simulink model "Charge_complete_V2"  (R2020a)
settings: Solver=VariableStepAuto  StartTime=0.0  StopTime=5500  RelTol=1e-3
undefined symbols (not defined in the file): Ion, Lithium
libraries: powerlib x7, electricdrivelib x1
settings Model: Creator=guill  LastModifiedBy=guill

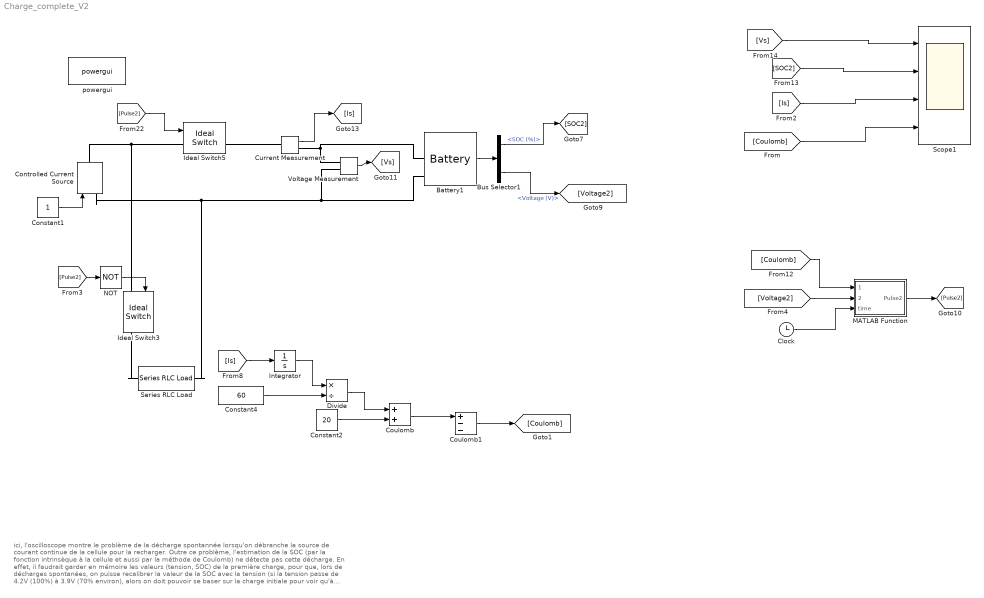
== system Charge_complete_V2 ==
  note: ici, l'oscilloscope montre le problème de la décharge spontannée lorsqu'on débranche la source de courant continue de la cellule pour la recharger. Outre ce problème, l'estimation de la SOC (par la fonction intrinsèque à la cellule et aussi par la méthode de Coulomb) ne détecte pas cette décharge.
      | En effet, il faudrait garder en mémoire les valeurs (tension, SOC) de la première charge, pour que, lors de décharges spontanées, on puisse recalibrer la valeur de la SOC avec la tension (si la tension passe de 4.2V (100%) à 3.9V (70% environ), alors on doit pouvoir se baser sur la charge initiale pour voir qu'à 3.9V, SOC=70%)
  Battery1 : electricdrivelib/Extra Sources/Battery  BatType=Lithium-Ion  ShowTempParam=on  ThermalPreset="3.6V  2.0Ah"  ShowAgeParam=off  NomV=3.5  NomQ=2  SOC=35  Batt_Tr=30  PresetModel=off  MaxQ=2.05  MinV=2.625  FullV=4.1  Dis_rate=0.4  R=0.017  Normal_OP=1.8087  expZone="[3.88         0.2]"  current=[6.5 13 32.5]  Units=Time  Tci=20  NomT=115  T2=0  MaxQ2=1.65  FullV2=4  Normal_OP2=3.25  expZone2="[3.8         0.2]"  Rca=0.06  ti=1000  Dp=0  Neq0=0  Tsim=1e6  Ta1=25  Qeol=5.4*0.9  Reol=0.013333*1.2  Char_age=[2.3478, 3]  Dis_age=[2.3478, 10]  N1=1500  N2=10500  N3=1000  N4=1400  Ta2=45  N5=950
  Bus Selector1 : BusSelector  OutputSignals=SOC (%),Current (A),Voltage (V)
  Clock : Clock
  Constant1 : Constant
  Constant2 : Constant  Value=20
  Constant4 : Constant  Value=60
  Controlled Current Source : powerlib/Electrical Sources/Controlled Current Source  Initialize=on  Source_Type=AC  Amplitude=0  Phase=0  Frequency=0  Measurements=None
  Coulomb : Sum
  Coulomb1 : Sum  Inputs=+--
  Current Measurement : powerlib/Measurements/Current Measurement  PhasorSimulation=off  OutputType=Complex  PSBequivalent=0
  Divide : Product  Inputs=*/
  Ideal Switch3 : powerlib/Power Electronics/Ideal Switch  Ron=0.001  Lon=0  IC=0  Rs=1e5  Cs=inf  Measurements=on
  Ideal Switch5 : powerlib/Power Electronics/Ideal Switch  Ron=0.001  Lon=0  IC=0  Rs=1e5  Cs=inf  Measurements=on
  Integrator : Integrator
  MATLAB Function : MATLAB Function  TreatAsAtomicUnit=on
  NOT : Logic  Operator=NOT  IconShape=distinctive  AllPortsSameDT=off  OutDataTypeStr=boolean
  Scope1 : Scope  NumInputPorts=4
  Series RLC Load : powerlib/Elements/Series RLC Load  LConnTagsString=a  RConnTagsString=__new0  NominalVoltage=10  NominalFrequency=60  ActivePower=1000  InductivePower=0  CapacitivePower=0  Setx0=off  InitialVoltage=0  SetiL0=off  InitialCurrent=0  Measurements=None  LoadType=constant Z
  Voltage Measurement : powerlib/Measurements/Voltage Measurement  PhasorSimulation=off  OutputType=Complex  PSBequivalent=0
  powergui : powerlib/powergui  Priority=1  SimulationMode=Continuous  SampleTime=50e-2  frequency=60  Iterations=50  frequencyindice=0  Pbase=100e6  ErrMax=1e-4  UnitsV=kV  UnitsW=MW  buscounter=0  FunctionMessages=off  echomessages=off  EnableUseOfTLC=off  CurrentSourceSwitches=off  DisableSnubberDevices=off  DisableRonSwitches=off  DisableVfSwitches=off  DisplayEquations=off  AutomaticDiscreteSolvers=off  SolverType=Tustin/Backward Euler (TBE)  Interpol=off  ExternalGateDelay=off  methode=off  Ts=100  x0status=blocks  SPID=on  SwTol=0  HookPort=off  NonlinearTolerance=1e-4  nMaxIteration=100  ContinueOnMaxIteration=off  RestoreLinks=warning  ResistiveCurrentMeasurement=off  Frange=[0:2:500]  Ylog=off  Xlog=on  ShowGrid=off  save=off  variable=ZData  structure=0  ZoomFFT=off  StartTime=0.0  cycles=1  DisplayStyle=1  fundamental=60  FreqAxis=off  MaxFrequency=1000  frequencyindicesteady=1  RmsSteady=1  display=off
  wires:
  [Is] -> Scope1/3
  Coulomb/1 -> Coulomb1/1
  Constant2/1 -> Coulomb/2
  [Pulse2] -> Ideal Switch5/1
  Bus Selector1/1 -> [SOC2]  "<SOC (%)>"
  Integrator/1 -> Divide/1
  Divide/1 -> Coulomb/1
  [SOC2] -> Scope1/2
  Constant1/1 -> Controlled Current Source/1
  NOT/1 -> Ideal Switch3/1
  Battery1/1 -> Bus Selector1/1
  Current Measurement/1 -> [Is]
  Bus Selector1/3 -> [Voltage2]  "<Voltage (V)>"
  [Pulse2] -> NOT/1
  [Coulomb] -> Scope1/4
  Constant4/1 -> Divide/2
  [Vs] -> Scope1/1
  Voltage Measurement/1 -> [Vs]
  [Is] -> Integrator/1
  Coulomb1/1 -> [Coulomb]
  MATLAB Function/1(Pulse2) -> [Pulse2]
  [Coulomb] -> MATLAB Function/1(Coulomb)
  [Voltage2] -> MATLAB Function/2(Voltage2)
  Clock/1 -> MATLAB Function/3(time)
  connections:
  Controlled Current Source/RConn1 -- Ideal Switch5/LConn1 -- Ideal Switch3/LConn1
  Controlled Current Source/LConn1 -- Battery1/LConn2 -- Voltage Measurement/LConn2 -- Series RLC Load/RConn1
  Current Measurement/RConn1 -- Battery1/LConn1 -- Voltage Measurement/LConn1
  Series RLC Load/LConn1 -- Ideal Switch3/RConn1
  Ideal Switch5/RConn1 -- Current Measurement/LConn1

== matlab function Charge_complete_V2/MATLAB Function ==
  data: Coulomb input; Pulse2 output; Voltage2 input; time input
function Pulse2 = fcn(Coulomb, Voltage2, time)
temps=[];
tension=[];
coulomb=[];
if Coulomb>100
    Pulse2=0;
else
    Pulse2=1;
end
%while Coulomb<100
  %  temps=[temps time];
   % coulomb=[coulomb Coulomb];
    %tension=[tension Voltage2];
%end
end
